simulink model "ESE4481NController"  (R2024a)
settings: Solver=VariableStepAuto  StartTime=0.0  StopTime=10.0  RelTol=1e-3
undefined symbols (not defined in the file): Jz, Kr, Kyaw, Yawc
settings Model: Creator=achic  LastModifiedBy=achic

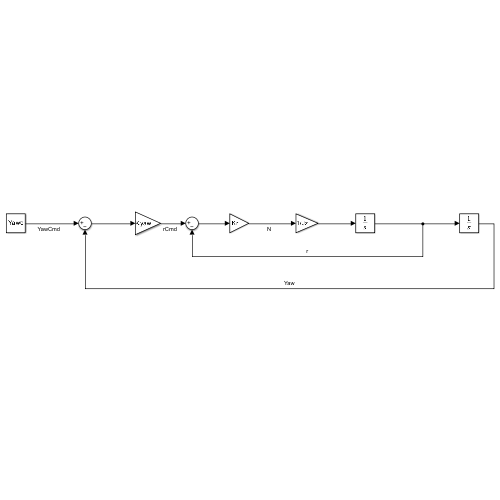
[thumbnail: Simulink's stored preview of the top-level diagram]
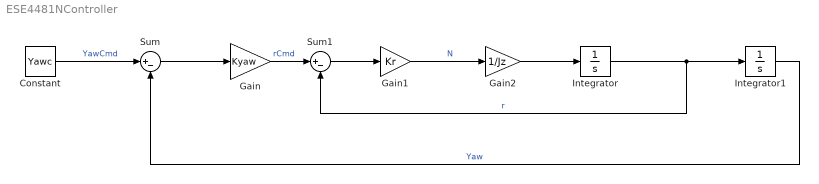
== system ESE4481NController ==
  Constant : Constant  Value=Yawc
  Gain : Gain  Gain=Kyaw
  Gain1 : Gain  Gain=Kr
  Gain2 : Gain  Gain=1/Jz
  Integrator : Integrator
  Integrator1 : Integrator
  Sum : Sum  Inputs=|+-
  Sum1 : Sum  Inputs=|+-
  wires:
  Gain2/1 -> Integrator/1
  Sum/1 -> Gain/1
  Sum1/1 -> Gain1/1
  Gain/1 -> Sum1/1  "rCmd"
  Integrator1/1 -> Sum/2  "Yaw"
  Gain1/1 -> Gain2/1  "N"
  Constant/1 -> Sum/1  "YawCmd"
  Integrator/1 -> Sum1/2, Integrator1/1  "r"
